simulink model "SemiOffline_Preprocessing_ECG"  (R2019a)
settings: Solver=FixedStepDiscrete  StartTime=0.0  StopTime=sim_time + param_frame_size_sec  FixedStep=1/fs  MaxStep=1/fs  RelTol=1e-3
undefined symbols (not defined in the file): fdesignblkfcn, fs, gcbh, param_frame_size_sec, tot_samples
(part 1 of 2)
settings Model: Creator=rcord  LastModifiedBy=rcord
settings DataIOCC: ExternalInput=[t, ecg]  LoadExternalInput=on
settings DebuggingCC: UnderSpecifiedDimensionMsg=warning

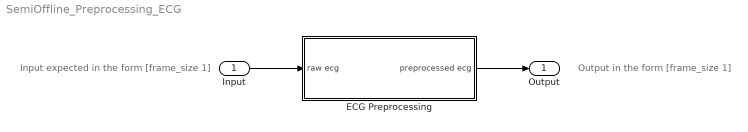
== system SemiOffline_Preprocessing_ECG ==
  note: Input expected in the form [frame_size 1]
  note: Output in the form [frame_size 1]
  Input : Inport  SampleTime=1/fs
  ECG Preprocessing : Subsystem  mask{param_ecg_gain_mv=1000, param_ecg_fc_lo=2.5, param_ecg_fc_hi=30, param_ecg_trans_bw=2}
      mask prompts: param_ecg_gain_mv "mV Conversion Gain"; param_ecg_fc_lo "Low Passband Frequency Corner (Hz)"; param_ecg_fc_hi "High Passband Frequency Corner (Hz)"; param_ecg_trans_bw "Transition bandwidth"
      mask init:
      | assignin('base','param_ecg_gain_mv',param_ecg_gain_mv)
      | assignin('base','param_ecg_fc_lo',param_ecg_fc_lo)
      | assignin('base','param_ecg_fc_hi',param_ecg_fc_hi)
      | assignin('base','param_ecg_trans_bw',param_ecg_trans_bw)
      mask DialogControl DescGroupVar Prompt: ECG Preprocessing
      mask DialogControl DescTextVar Prompt: Preprocessing of the ECG. This involves an amplificaiton stage followed by a filtfiltering operation (i.e. a front-back zero-phase FIR bandpass filter).
  Output : Outport
  wires:
  Input/1 -> ECG Preprocessing/1(raw ecg)
  ECG Preprocessing/1(preprocessed ecg) -> Output/1

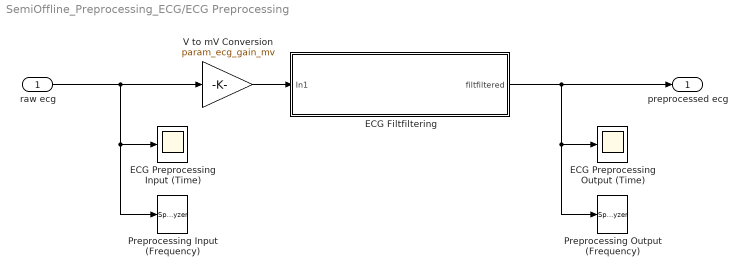
== system SemiOffline_Preprocessing_ECG/ECG Preprocessing ==
  raw ecg : Inport
  ECG Filtfiltering : Subsystem
  ECG Preprocessing Input (Time) : Scope
  ECG Preprocessing Output (Time) : Scope
  Preprocessing Input (Frequency) : SpectrumAnalyzer
  Preprocessing Output (Frequency) : SpectrumAnalyzer
  V to mV Conversion : Gain  Gain=param_ecg_gain_mv
  preprocessed ecg : Outport
  wires:
  ECG Filtfiltering/1(filtfiltered) -> preprocessed ecg/1, ECG Preprocessing Output (Time)/1, Preprocessing Output (Frequency)/1
  raw ecg/1 -> Preprocessing Input (Frequency)/1, ECG Preprocessing Input (Time)/1, V to mV Conversion/1
  V to mV Conversion/1 -> ECG Filtfiltering/1(In1)

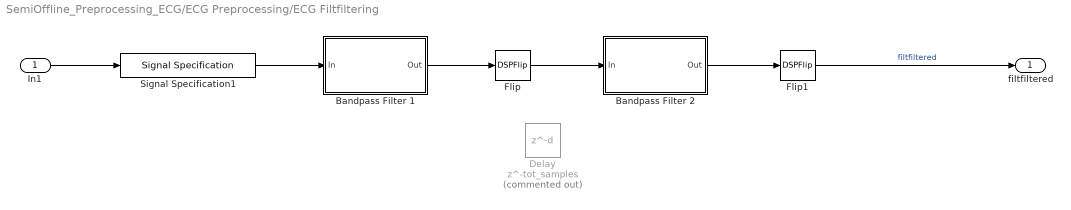
== system SemiOffline_Preprocessing_ECG/ECG Preprocessing/ECG Filtfiltering ==
  In1 : Inport
  Bandpass Filter 1 : Subsystem  DialogController=fdesignblkfcn  InitFcn=fdesignblkfcn(gcbh, {'InitFcn'});  mask(Bandpass Filter){}
      mask help: Design a bandpass filter
      settings: CopyFcn=fdesignblkfcn(gcbh, {'CopyFcn'});
      mask Help: helpview(mapfilelocation('dsp'), 'dspbandpassfilter');
      mask Display: disp('Bandpass');
  Bandpass Filter 2 : Subsystem  DialogController=fdesignblkfcn  InitFcn=fdesignblkfcn(gcbh, {'InitFcn'});  mask(Bandpass Filter){}
      mask help: Design a bandpass filter
      settings: CopyFcn=fdesignblkfcn(gcbh, {'CopyFcn'});
      mask Help: helpview(mapfilelocation('dsp'), 'dspbandpassfilter');
      mask Display: disp('Bandpass');
  Delay : Delay  Commented=on  DelayLength=tot_samples
  Flip : DSPFlip
  Flip1 : DSPFlip
  Signal Specification1 : SignalSpecification  Dimensions=[param_frame_size_sec*fs 1]
  filtfiltered : Outport
  wires:
  Flip/1 -> Bandpass Filter 2/1(In)
  Signal Specification1/1 -> Bandpass Filter 1/1(In)
  Flip1/1 -> filtfiltered/1  "filtfiltered"
  Bandpass Filter 1/1(Out) -> Flip/1
  In1/1 -> Signal Specification1/1
  Bandpass Filter 2/1(Out) -> Flip1/1

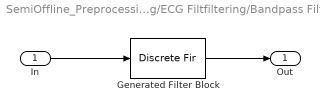
== system SemiOffline_Preprocessing_ECG/ECG Preprocessing/ECG Filtfiltering/Bandpass Filter 1 ==
  In : Inport
  Generated Filter Block : DiscreteFir  Tag=BlockMethodSubSystem  Coefficients=[-0.000604978320771744826 -0.000235083115883526813 -0.000273530821723848056 -0.000310443121022179402 -0.000345055215889066046 -0.000375510837104244769 -0.00040049209394480464 -0.00041780425523977601 -0.000426552548350842833 -0.000425344657371441433 -0.000413527419470029959 -0.000388558631828530199 -0.000350359211139658502 -0.000299745411776331265 -0.000234311692324289979 -0.000156055496166101907 -6.44249053728080745e-05 3.94344245054481296e-05 0.000154281756394008933 0.000278323414132151936 0.000409574862434147595 0.000545953678508312532 0.000684757122602292932 0.000823030568979907663 0.000958113018864269325 0.00108706186227524758 0.00120649217897672166 0.00131426927590056614 0.00140691726742189251 0.00148246012177367394 0.00153829272159941447 0.00157307929085900725 0.00158509340368087961 0.00157380333902921868 0.00153867078167277643 0.00148031079880637248 0.00139912661302633704 0.00129706232030104142 0.00117565377839331121 0.00103753424382136902 0.000885499651109533897 0.000722903061455593219 0.000553168576781724961 0.000380155303215198252 0.000207569854859765445 3.93888806664771446e-05 -0.000120882309211992165 -0.000269496855109876228 -0.000403449946450762712 -0.000519887228019691797 -0.000616563080471777773 -0.000691606985101301088 -0.000744080741767522234 -0.000773220171352047812 -0.00077945069638684695 -0.000763298224089631436 -0.000726467115048749887 -0.000670635252979840573 -0.000598571169442946652 -0.000512987774384702101 -0.000417368713296364404 -0.00031495114730563465 -0.000209693686967796287 -0.000104902728834760156 -4.44690680818200183e-06 8.85925327654278789e-05 0.000170950737728648252 0.000240252658976125339 0.000294166342470323532 0.000331311830754013961 0.000350555761692395199 0.000351787261201512512 0.000335094178143251155 0.00030166451466417829 0.000252840591756254673 0.000190846316699891459 0.000118083056019187066 3.76162884349192598e-05 -4.75447700928875207e-05 -0.00013389708250264497 -0.000218251353464577141 -0.000297109418525390171 -0.000367592828494043254 -0.000426667616853404822 -0.000472131177326803669 -0.000501884108192684271 -0.000514729653652615769 -0.000509677328207022696 -0.000486810620621723673 -0.000446369531931162483 -0.000389692917314981863 -0.000318223530700122701 -0.000234394770684352998 -0.000140618004409548099 -4.00904349968857925e-05 6.41295668775877402e-05 0.000168491614234262841 0.000269821774158510901 0.0003646356182697063 0.000450104577847115913 0.000523334549393006648 0.00058222990572613252 0.000624878475009158461 0.000650277541892643599 0.000657733932393517076 0.000647494048306962466 0.000620157400677535833 0.000577262943489921109 0.000520571454599278631 0.00045270612430950419 0.000376370421040053303 0.000294886564188957009 0.000211484911465107989 0.000129782935909014728 5.30198679591795336e-05 -1.54035689324979433e-05 -7.27239120254416743e-05 -0.000116214755286621124 -0.000144028241031264321 -0.000154510275227954152 -0.000146996760733282344 -0.000121164727865655166 -7.76856996630245918e-05 -1.75590793113062195e-05 5.72361027383123293e-05 0.000144509761683518146 0.000241248723796134903 0.000344392120245392533 0.000450291282341344439 0.000555468698704171277 0.000656155536322569101 0.000748967767418521864 0.000830526955355782165 0.000898105715880628493 0.000949177359661756916 0.000982080009962424741 0.000995535352843296114 0.000989216272556177941 0.000963271590154880938 0.000918812707506674745 0.000857393844717917273 0.000781435362468952234 0.000693662814810993688 0.00059751917759335259 0.000496493510598246821 0.000394557130295916279 0.000295474957389456826 0.000203179398476785315 0.000121128926042667268 5.26822387366519969e-05 4.49600295923560482e-07 -3.3282412096467557e-05 -4.71659293415656712e-05 -4.03130834101184305e-05 -1.2880948430750059e-05 3.44605600059980002e-05 0.000100047110162757632 0.000181730761162674946 0.000276520015434537263 0.000381123513109075441 0.000491613542897385587 0.000604018106592785166 0.000714032576360607105 0.000817596831607618566 0.000910637435132874667 ...(+20190 chars)]  InputProcessing=Columns as channels (frame based)
  Out : Outport
  wires:
  In/1 -> Generated Filter Block/1
  Generated Filter Block/1 -> Out/1
